simulink model "s_cd_hmc_v3_pol0"  (R2016b)
(part 2 of 31)

      | port_label('output', 1, 'q');
      | disp(['Z^-', num2str(latency)]);
  pipeline92 : Subsystem  AncestorBlock=casper_library_delays/pipeline  mask(pipeline){latency=1}
      mask help:
      | An explicitly laid-out delay line to avoid mapping to SRL16s
      | for use in pipelining to help achieve timing closure.
      mask init:
      | pipeline_init(gcb,'latency',latency);
      settings: AttributesFormatString=Latency = %<latency>
      mask Display:
      | port_label('input', 1, 'd');
      | port_label('output', 1, 'q');
      | disp(['Z^-', num2str(latency)]);
  pipeline93 : Subsystem  AncestorBlock=casper_library_delays/pipeline  mask(pipeline){latency=1}
      mask help:
      | An explicitly laid-out delay line to avoid mapping to SRL16s
      | for use in pipelining to help achieve timing closure.
      mask init:
      | pipeline_init(gcb,'latency',latency);
      settings: AttributesFormatString=Latency = %<latency>
      mask Display:
      | port_label('input', 1, 'd');
      | port_label('output', 1, 'q');
      | disp(['Z^-', num2str(latency)]);
  pipeline94 : Subsystem  AncestorBlock=casper_library_delays/pipeline  mask(pipeline){latency=1}
      mask help:
      | An explicitly laid-out delay line to avoid mapping to SRL16s
      | for use in pipelining to help achieve timing closure.
      mask init:
      | pipeline_init(gcb,'latency',latency);
      settings: AttributesFormatString=Latency = %<latency>
      mask Display:
      | port_label('input', 1, 'd');
      | port_label('output', 1, 'q');
      | disp(['Z^-', num2str(latency)]);
  pipeline95 : Subsystem  AncestorBlock=casper_library_delays/pipeline  mask(pipeline){latency=1}
      mask help:
      | An explicitly laid-out delay line to avoid mapping to SRL16s
      | for use in pipelining to help achieve timing closure.
      mask init:
      | pipeline_init(gcb,'latency',latency);
      settings: AttributesFormatString=Latency = %<latency>
      mask Display:
      | port_label('input', 1, 'd');
      | port_label('output', 1, 'q');
      | disp(['Z^-', num2str(latency)]);
  pipeline96 : Subsystem  AncestorBlock=casper_library_delays/pipeline  mask(pipeline){latency=1}
      mask help:
      | An explicitly laid-out delay line to avoid mapping to SRL16s
      | for use in pipelining to help achieve timing closure.
      mask init:
      | pipeline_init(gcb,'latency',latency);
      settings: AttributesFormatString=Latency = %<latency>
      mask Display:
      | port_label('input', 1, 'd');
      | port_label('output', 1, 'q');
      | disp(['Z^-', num2str(latency)]);
  pipeline97 : Subsystem  AncestorBlock=casper_library_delays/pipeline  mask(pipeline){latency=1}
      mask help:
      | An explicitly laid-out delay line to avoid mapping to SRL16s
      | for use in pipelining to help achieve timing closure.
      mask init:
      | pipeline_init(gcb,'latency',latency);
      settings: AttributesFormatString=Latency = %<latency>
      mask Display:
      | port_label('input', 1, 'd');
      | port_label('output', 1, 'q');
      | disp(['Z^-', num2str(latency)]);
  pipeline98 : Subsystem  AncestorBlock=casper_library_delays/pipeline  mask(pipeline){latency=1}
      mask help:
      | An explicitly laid-out delay line to avoid mapping to SRL16s
      | for use in pipelining to help achieve timing closure.
      mask init:
      | pipeline_init(gcb,'latency',latency);
      settings: AttributesFormatString=Latency = %<latency>
      mask Display:
      | port_label('input', 1, 'd');
      | port_label('output', 1, 'q');
      | disp(['Z^-', num2str(latency)]);
  pipeline99 : Subsystem  AncestorBlock=casper_library_delays/pipeline  mask(pipeline){latency=2}
      mask help:
      | An explicitly laid-out delay line to avoid mapping to SRL16s
      | for use in pipelining to help achieve timing closure.
      mask init:
      | pipeline_init(gcb,'latency',latency);
      settings: AttributesFormatString=Latency = %<latency>
      mask Display:
      | port_label('input', 1, 'd');
      | port_label('output', 1, 'q');
      | disp(['Z^-', num2str(latency)]);
  port0 : Subsystem  Tag=xps:sw_reg  AncestorBlock=xps_library/software register  mask(swreg){io_dir=From Processor, io_delay=0, sample_period=1, names=reg, bitwidths=32, bin_pts=0, arith_types=0, sim_port=on, show_format=on}
      mask prompts: io_dir "I/O direction"; io_delay "I/O delay"; sample_period "Sample period"; names "Bitfield names [msb...lsb]"; bitwidths "Bitfield widths"; bin_pts "Bitfield binary pts"; arith_types "Bitfield types, ufix=0, fix=1, bool=2"; sim_port "Provide sim input/output?"; show_format "Print format string?"
      mask help: A 32-bit software-accessible register. Can be divided into bitfields of varying widths and types using the fields in the block mask.
      mask init:
      | swreg_init(gcb)
      settings: AttributesFormatString=1input:uf32.0 = 32 bits
      mask TypeOptions io_dir: To Processor | From Processor
      mask Callback io_dir:
      | mask_enables = get_param(gcb, 'MaskEnables');
      | mask_names = get_param(gcb, 'MaskNames');
      | if strcmp(get_param(gcb, 'io_dir'), 'To Processor'),
      |     mask_enables{ismember(mask_names, 'sample_period')} = 'off';
      | else
      |     mask_enables{ismember(mask_names, 'sample_period')} = 'on';
      | end
      | set_param(gcb, 'MaskEnables', mask_enables);
  sync : Subsystem  Tag=xps:sw_reg  AncestorBlock=xps_library/software_register  mask(swreg){io_dir=To Processor, io_delay=0, sample_period=1, names=reg, bitwidths=1, bin_pts=0, arith_types=2, sim_port=on, show_format=on}
      mask prompts: io_dir "I/O direction"; io_delay "I/O delay"; sample_period "Sample period"; names "Bitfield names [msb...lsb]"; bitwidths "Bitfield widths"; bin_pts "Bitfield binary pts"; arith_types "Bitfield types, ufix=0, fix=1, bool=2"; sim_port "Provide sim input/output?"; show_format "Print format string?"
      mask help: A 32-bit software-accessible register. Can be divided into bitfields of varying widths and types using the fields in the block mask.
      mask init:
      | swreg_init(gcb)
      settings: AttributesFormatString=1output:b = 1 bits
      mask TypeOptions io_dir: To Processor | From Processor
      mask Callback io_dir:
      | mask_enables = get_param(gcb, 'MaskEnables');
      | mask_names = get_param(gcb, 'MaskNames');
      | if strcmp(get_param(gcb, 'io_dir'), 'To Processor'),
      |     mask_enables{ismember(mask_names, 'sample_period')} = 'off';
      | else
      |     mask_enables{ismember(mask_names, 'sample_period')} = 'on';
      | end
      | set_param(gcb, 'MaskEnables', mask_enables);
  sync_cnt : Subsystem  Tag=xps:sw_reg  AncestorBlock=xps_library/software_register  mask(swreg){io_dir=To Processor, io_delay=0, sample_period=1, names=reg, bitwidths=32, bin_pts=0, arith_types=0, sim_port=on, show_format=on}
      mask prompts: io_dir "I/O direction"; io_delay "I/O delay"; sample_period "Sample period"; names "Bitfield names [msb...lsb]"; bitwidths "Bitfield widths"; bin_pts "Bitfield binary pts"; arith_types "Bitfield types, ufix=0, fix=1, bool=2"; sim_port "Provide sim input/output?"; show_format "Print format string?"
      mask help: A 32-bit software-accessible register. Can be divided into bitfields of varying widths and types using the fields in the block mask.
      mask init:
      | swreg_init(gcb)
      settings: AttributesFormatString=1output:uf32.0 = 32 bits
      mask TypeOptions io_dir: To Processor | From Processor
      mask Callback io_dir:
      | mask_enables = get_param(gcb, 'MaskEnables');
      | mask_names = get_param(gcb, 'MaskNames');
      | if strcmp(get_param(gcb, 'io_dir'), 'To Processor'),
      |     mask_enables{ismember(mask_names, 'sample_period')} = 'off';
      | else
      |     mask_enables{ismember(mask_names, 'sample_period')} = 'on';
      | end
      | set_param(gcb, 'MaskEnables', mask_enables);
  sync_select : Subsystem  Tag=xps:sw_reg  AncestorBlock=xps_library/software register  mask(swreg){io_dir=From Processor, io_delay=0, sample_period=1, names=reg, bitwidths=2, bin_pts=0, arith_types=0, sim_port=on, show_format=on}
      mask prompts: io_dir "I/O direction"; io_delay "I/O delay"; sample_period "Sample period"; names "Bitfield names [msb...lsb]"; bitwidths "Bitfield widths"; bin_pts "Bitfield binary pts"; arith_types "Bitfield types, ufix=0, fix=1, bool=2"; sim_port "Provide sim input/output?"; show_format "Print format string?"
      mask help: A 32-bit software-accessible register. Can be divided into bitfields of varying widths and types using the fields in the block mask.
      mask init:
      | swreg_init(gcb)
      settings: AttributesFormatString=1input:uf2.0 = 2 bits
      mask TypeOptions io_dir: To Processor | From Processor
      mask Callback io_dir:
      | mask_enables = get_param(gcb, 'MaskEnables');
      | mask_names = get_param(gcb, 'MaskNames');
      | if strcmp(get_param(gcb, 'io_dir'), 'To Processor'),
      |     mask_enables{ismember(mask_names, 'sample_period')} = 'off';
      | else
      |     mask_enables{ismember(mask_names, 'sample_period')} = 'on';
      | end
      | set_param(gcb, 'MaskEnables', mask_enables);
  time_gen_cd : Subsystem  mask{n_bits_period=fft_stages-1-2, n_bits_increment=0, n_bits_counter=48-fft_stages}
      mask prompts: n_bits_period "Period (2^?)"; n_bits_increment "Increment (2^?)"; n_bits_counter "Counter size (2^?)"
  tl_cd0 : Subsystem  mask(timed_latch){n_bits_time=48-fft_stages, n_bits_quantization=fft_stages, n_bits_counters=4}
      mask prompts: n_bits_time "Number bits in time to compare"; n_bits_quantization "Time offset from lsb"; n_bits_counters "Bits in status counters"
      mask help:
      | Latches load_value when armed and current_time matches requested time.
      | current_time should be in ADC samples.
      mask init:
      | set_param([gcb,'/status'], 'bitwidths', mat2str([1, repmat(n_bits_counters, 1, 2)]));
      mask Help:
      | When armed, will latch new value when current time matches the time
      | specified. The input time should be in samples and mask settings allow
      | a portion of this to be compared to cater for quantization. Arm and latch
      | counts allow the current state, pending and missed latch events to be
      | determined.
  tl_cd0_control : Subsystem  Tag=xps:sw_reg  AncestorBlock=xps_library/software_register  mask(swreg){io_dir=From Processor, io_delay=0, sample_period=1, names=[arm load_immediate load_time_msw], bitwidths=[1 1 16], bin_pts=[0 0 0], arith_types=[2 2 0], sim_port=on, show_format=on}
      mask prompts: io_dir "I/O direction"; io_delay "I/O delay"; sample_period "Sample period"; names "Bitfield names [msb...lsb]"; bitwidths "Bitfield widths"; bin_pts "Bitfield binary pts"; arith_types "Bitfield types, ufix=0, fix=1, bool=2"; sim_port "Provide sim input/output?"; show_format "Print format string?"
      mask help: A 32-bit software-accessible register. Can be divided into bitfields of varying widths and types using the fields in the block mask.
      mask init:
      | swreg_init(gcb)
      settings: AttributesFormatString=3 inputs:b,b,uf16.0 = 18 bits
      mask TypeOptions io_dir: To Processor | From Processor
      mask Callback io_dir:
      | mask_enables = get_param(gcb, 'MaskEnables');
      | mask_names = get_param(gcb, 'MaskNames');
      | if strcmp(get_param(gcb, 'io_dir'), 'To Processor'),
      |     mask_enables{ismember(mask_names, 'sample_period')} = 'off';
      | else
      |     mask_enables{ismember(mask_names, 'sample_period')} = 'on';
      | end
      | set_param(gcb, 'MaskEnables', mask_enables);
  tl_cd0_control_lsw : Subsystem  Tag=xps:sw_reg  AncestorBlock=xps_library/software_register  mask(swreg){io_dir=From Processor, io_delay=0, sample_period=1, names=load_time_lsw, bitwidths=32, bin_pts=0, arith_types=0, sim_port=on, show_format=on}
      mask prompts: io_dir "I/O direction"; io_delay "I/O delay"; sample_period "Sample period"; names "Bitfield names [msb...lsb]"; bitwidths "Bitfield widths"; bin_pts "Bitfield binary pts"; arith_types "Bitfield types, ufix=0, fix=1, bool=2"; sim_port "Provide sim input/output?"; show_format "Print format string?"
      mask help: A 32-bit software-accessible register. Can be divided into bitfields of varying widths and types using the fields in the block mask.
      mask init:
      | swreg_init(gcb)
      settings: AttributesFormatString=1input:uf32.0 = 32 bits
      mask TypeOptions io_dir: To Processor | From Processor
      mask Callback io_dir:
      | mask_enables = get_param(gcb, 'MaskEnables');
      | mask_names = get_param(gcb, 'MaskNames');
      | if strcmp(get_param(gcb, 'io_dir'), 'To Processor'),
      |     mask_enables{ismember(mask_names, 'sample_period')} = 'off';
      | else
      |     mask_enables{ismember(mask_names, 'sample_period')} = 'on';
      | end
      | set_param(gcb, 'MaskEnables', mask_enables);
  tl_cd1_control : Subsystem  Tag=xps:sw_reg  AncestorBlock=xps_library/software_register  mask(swreg){io_dir=From Processor, io_delay=0, sample_period=1, names=[arm load_immediate load_time_msw], bitwidths=[1 1 16], bin_pts=[0 0 0], arith_types=[2 2 0], sim_port=on, show_format=on}
      mask prompts: io_dir "I/O direction"; io_delay "I/O delay"; sample_period "Sample period"; names "Bitfield names [msb...lsb]"; bitwidths "Bitfield widths"; bin_pts "Bitfield binary pts"; arith_types "Bitfield types, ufix=0, fix=1, bool=2"; sim_port "Provide sim input/output?"; show_format "Print format string?"
      mask help: A 32-bit software-accessible register. Can be divided into bitfields of varying widths and types using the fields in the block mask.
      mask init:
      | swreg_init(gcb)
      settings: AttributesFormatString=3 inputs:b,b,uf16.0 = 18 bits
      mask TypeOptions io_dir: To Processor | From Processor
      mask Callback io_dir:
      | mask_enables = get_param(gcb, 'MaskEnables');
      | mask_names = get_param(gcb, 'MaskNames');
      | if strcmp(get_param(gcb, 'io_dir'), 'To Processor'),
      |     mask_enables{ismember(mask_names, 'sample_period')} = 'off';
      | else
      |     mask_enables{ismember(mask_names, 'sample_period')} = 'on';
      | end
      | set_param(gcb, 'MaskEnables', mask_enables);
  tl_cd1_control_lsw : Subsystem  Tag=xps:sw_reg  AncestorBlock=xps_library/software_register  mask(swreg){io_dir=From Processor, io_delay=0, sample_period=1, names=load_time_lsw, bitwidths=32, bin_pts=0, arith_types=0, sim_port=on, show_format=on}
      mask prompts: io_dir "I/O direction"; io_delay "I/O delay"; sample_period "Sample period"; names "Bitfield names [msb...lsb]"; bitwidths "Bitfield widths"; bin_pts "Bitfield binary pts"; arith_types "Bitfield types, ufix=0, fix=1, bool=2"; sim_port "Provide sim input/output?"; show_format "Print format string?"
      mask help: A 32-bit software-accessible register. Can be divided into bitfields of varying widths and types using the fields in the block mask.
      mask init:
      | swreg_init(gcb)
      settings: AttributesFormatString=1input:uf32.0 = 32 bits
      mask TypeOptions io_dir: To Processor | From Processor
      mask Callback io_dir:
      | mask_enables = get_param(gcb, 'MaskEnables');
      | mask_names = get_param(gcb, 'MaskNames');
      | if strcmp(get_param(gcb, 'io_dir'), 'To Processor'),
      |     mask_enables{ismember(mask_names, 'sample_period')} = 'off';
      | else
      |     mask_enables{ismember(mask_names, 'sample_period')} = 'on';
      | end
      | set_param(gcb, 'MaskEnables', mask_enables);
  tl_cd_bs0 : Subsystem  mask(timed_latch){n_bits_time=48-fft_stages, n_bits_quantization=fft_stages, n_bits_counters=4}
      mask prompts: n_bits_time "Number bits in time to compare"; n_bits_quantization "Time offset from lsb"; n_bits_counters "Bits in status counters"
      mask help:
      | Latches load_value when armed and current_time matches requested time.
      | current_time should be in ADC samples.
      mask init:
      | set_param([gcb,'/status'], 'bitwidths', mat2str([1, repmat(n_bits_counters, 1, 2)]));
      mask Help:
      | When armed, will latch new value when current time matches the time
      | specified. The input time should be in samples and mask settings allow
      | a portion of this to be compared to cater for quantization. Arm and latch
      | counts allow the current state, pending and missed latch events to be
      | determined.
  tx_metadata : Subsystem  Tag=xps:sw_reg  AncestorBlock=xps_library/software register  mask(swreg){io_dir=From Processor, io_delay=0, sample_period=1, names=[porttx board_id], bitwidths=16, bin_pts=0, arith_types=0, sim_port=on, show_format=on}
      mask prompts: io_dir "I/O direction"; io_delay "I/O delay"; sample_period "Sample period"; names "Bitfield names [msb...lsb]"; bitwidths "Bitfield widths"; bin_pts "Bitfield binary pts"; arith_types "Bitfield types, ufix=0, fix=1, bool=2"; sim_port "Provide sim input/output?"; show_format "Print format string?"
      mask help: A 32-bit software-accessible register. Can be divided into bitfields of varying widths and types using the fields in the block mask.
      mask init:
      | swreg_init(gcb)
      settings: AttributesFormatString=2 inputs:uf16.0,uf16.0 = 32 bits
      mask TypeOptions io_dir: To Processor | From Processor
      mask Callback io_dir:
      | mask_enables = get_param(gcb, 'MaskEnables');
      | mask_names = get_param(gcb, 'MaskNames');
      | if strcmp(get_param(gcb, 'io_dir'), 'To Processor'),
      |     mask_enables{ismember(mask_names, 'sample_period')} = 'off';
      | else
      |     mask_enables{ismember(mask_names, 'sample_period')} = 'on';
      | end
      | set_param(gcb, 'MaskEnables', mask_enables);
  valid80 : Subsystem  Tag=xps:sw_reg  AncestorBlock=xps_library/software_register  mask(swreg){io_dir=To Processor, io_delay=0, sample_period=1, names=reg, bitwidths=1, bin_pts=0, arith_types=2, sim_port=on, show_format=on}
      mask prompts: io_dir "I/O direction"; io_delay "I/O delay"; sample_period "Sample period"; names "Bitfield names [msb...lsb]"; bitwidths "Bitfield widths"; bin_pts "Bitfield binary pts"; arith_types "Bitfield types, ufix=0, fix=1, bool=2"; sim_port "Provide sim input/output?"; show_format "Print format string?"
      mask help: A 32-bit software-accessible register. Can be divided into bitfields of varying widths and types using the fields in the block mask.
      mask init:
      | swreg_init(gcb)
      settings: AttributesFormatString=1output:b = 1 bits
      mask TypeOptions io_dir: To Processor | From Processor
      mask Callback io_dir:
      | mask_enables = get_param(gcb, 'MaskEnables');
      | mask_names = get_param(gcb, 'MaskNames');
      | if strcmp(get_param(gcb, 'io_dir'), 'To Processor'),
      |     mask_enables{ismember(mask_names, 'sample_period')} = 'off';
      | else
      |     mask_enables{ismember(mask_names, 'sample_period')} = 'on';
      | end
      | set_param(gcb, 'MaskEnables', mask_enables);
  valid80_cnt : Subsystem  Tag=xps:sw_reg  AncestorBlock=xps_library/software_register  mask(swreg){io_dir=To Processor, io_delay=0, sample_period=1, names=reg, bitwidths=32, bin_pts=0, arith_types=0, sim_port=on, show_format=on}
      mask prompts: io_dir "I/O direction"; io_delay "I/O delay"; sample_period "Sample period"; names "Bitfield names [msb...lsb]"; bitwidths "Bitfield widths"; bin_pts "Bitfield binary pts"; arith_types "Bitfield types, ufix=0, fix=1, bool=2"; sim_port "Provide sim input/output?"; show_format "Print format string?"
      mask help: A 32-bit software-accessible register. Can be divided into bitfields of varying widths and types using the fields in the block mask.
      mask init:
      | swreg_init(gcb)
      settings: AttributesFormatString=1output:uf32.0 = 32 bits
      mask TypeOptions io_dir: To Processor | From Processor
      mask Callback io_dir:
      | mask_enables = get_param(gcb, 'MaskEnables');
      | mask_names = get_param(gcb, 'MaskNames');
      | if strcmp(get_param(gcb, 'io_dir'), 'To Processor'),
      |     mask_enables{ismember(mask_names, 'sample_period')} = 'off';
      | else
      |     mask_enables{ismember(mask_names, 'sample_period')} = 'on';
      | end
      | set_param(gcb, 'MaskEnables', mask_enables);
  wb_prog_delay : Subsystem  mask{n_bits_fft=fft_stages, n_bits_cd=17}
      mask prompts: n_bits_fft "fft length (2^?)"; n_bits_cd "max coarse delay (2^?)"
  tag scope: addr_map_sel=global, cnt_rst=global, dvalid=global, sync_select=global, sys_rst=global
  wires:
  Constant/1 -> port0/1(sim_1)
  port0/1(in_reg) -> Delay16/1
  Constant2/1 -> ip0/1(sim_1)
  ip0/1(in_reg) -> Delay15/1
  Constant3/1 -> forty_gbe/8(rx_overrun_ack)
  Constant4/1 -> forty_gbe/7(rx_ack)
  [gbe_rst] -> pipeline102/1(d)
  Delay15/1 -> forty_gbe/4(tx_dest_ip)
  Delay16/1 -> forty_gbe/5(tx_dest_port)
  Concat22/1 -> pipeline29/1(d)
  Concat3/1 -> pipeline27/1(d)
  phase0/1(in_initial) -> Reinterpret2/1
  delta_delay0/1(in_delta) -> Reinterpret1/1
  phase0/2(in_delta) -> Reinterpret3/1
  Reinterpret8/1 -> pipeline56/1(d)
  Reinterpret1/1 -> pipeline55/1(d)
  Reinterpret2/1 -> pipeline54/1(d)
  Reinterpret3/1 -> pipeline53/1(d)
  phase1/1(in_initial) -> Reinterpret5/1
  delta_delay1/1(in_delta) -> Reinterpret4/1
  phase1/2(in_delta) -> Reinterpret6/1
  Reinterpret4/1 -> pipeline51/1(d)
  Reinterpret5/1 -> pipeline50/1(d)
  Reinterpret6/1 -> pipeline49/1(d)
  Reinterpret7/1 -> pipeline52/1(d)
  delay0/1(in_initial) -> Reinterpret8/1
  delay1/1(in_initial) -> Reinterpret7/1
  Constant10/1 -> iptx_base/1(sim_1)
  Constant9/1 -> tx_metadata/1(sim_1)
  Constant13/1 -> tx_metadata/2(sim_2)
  iptx_base/1(in_reg) -> pipeline105/1(d)
  pipeline105/1(q) -> [tx_ip_base]
  tx_metadata/1(in_porttx) -> pipeline106/1(d)
  tx_metadata/2(in_board_id) -> pipeline107/1(d)
  pipeline106/1(q) -> [tx_port]
  pipeline107/1(q) -> [tx_board_id]
  edge_detect4/1(out) -> pipeline5/1(d)
  control/6(in_cnt_rst) -> edge_detect1/1(in)
  edge_detect1/1(out) -> pipeline14/1(d)
  control/3(in_gbe_rst) -> pipeline6/1(d)
  control/1(in_sys_rst) -> edge_detect7/1(in)
  pipeline3/1(q) -> [sys_rst]
  pipeline5/1(q) -> [clr_status]
  pipeline6/1(q) -> [gbe_rst]
  pipeline7/1(q) -> [gbe_txen]
  pipeline13/1(q) -> [tvg_adc_en]
  pipeline14/1(q) -> [cnt_rst]
  control/5(in_tvg_adc) -> pipeline13/1(d)
  edge_detect2/1(out) -> pipeline38/1(d)
  pipeline38/1(q) -> [gbe_cnt_rst]
  control/7(in_gbe_cnt_rst) -> edge_detect2/1(in)
  control/4(in_gbe_txen) -> pipeline7/1(d)
  control/2(in_status_clr) -> edge_detect4/1(in)
  pipeline43/1(q) -> [adc_snap_arm]
  control/8(in_adc_snap_arm) -> pipeline43/1(d)
  control/9(in_adc_snap_trig_select) -> pipeline39/1(d)
  pipeline39/1(q) -> [adc_snap_trig_source]
  Counter2/1 -> pipeline31/1(d)
  Counter4/1 -> pipeline32/1(d)
  Counter9/1 -> pipeline33/1(d)
  Counter10/1 -> pipeline34/1(d)
  Counter11/1 -> pipeline35/1(d)
  Counter12/1 -> pipeline36/1(d)
  Counter14/1 -> pipeline40/1(d)
  Counter13/1 -> pipeline37/1(d)
  hmc_error/1(sim_out) -> Terminator9/1
  [hmc_error] -> hmc_error/1(out_reg)
  hmc_parity/1(sim_out) -> Terminator11/1
  [hmc_parity_pol0] -> hmc_parity/1(out_reg)
  Constant11/1 -> Delay10/1
  [valid80_local] -> Gateway Out19/1, pipeline58/1(d), pipeline61/1(d), pipeline62/1(d), pipeline63/1(d), pipeline64/1(d), pipeline65/1(d), pipeline66/1(d), pipeline60/1(d), pipeline59/1(d)
  bus_create1/1(bus_out) -> [cd_in]
  pipeline30/1(q) -> [valid80_cd]
  Constant24/1 -> forty_gbe/2(tx_data)
  Constant25/1 -> forty_gbe/3(tx_valid)
  Constant26/1 -> forty_gbe/6(tx_end_of_frame)
  pipeline27/1(q) -> [ld_val1]
  pipeline29/1(q) -> [ld_val0]
  pipeline49/1(q) -> Concat3/4
  pipeline50/1(q) -> Concat3/3
  pipeline51/1(q) -> Concat3/2
  pipeline52/1(q) -> Concat3/1
  pipeline53/1(q) -> Concat22/4
  pipeline54/1(q) -> Concat22/3
  pipeline55/1(q) -> Concat22/2
  pipeline56/1(q) -> Concat22/1
  bus_expand2/1(msb_out8) -> pipeline167/1(d)  "hmc_out9"
  bus_expand2/8(lsb_out1) -> pipeline73/1(d)  "hmc_out16"
  pipeline73/1(q) -> hmc_out/8(in_d07)
  pipeline72/1(q) -> hmc_out/7(in_d06)
  pipeline71/1(q) -> hmc_out/6(in_d05)
  pipeline70/1(q) -> hmc_out/5(in_d04)
  pipeline69/1(q) -> hmc_out/4(in_d03)
  pipeline68/1(q) -> hmc_out/3(in_d02)
  pipeline67/1(q) -> hmc_out/2(in_d01)
  pipeline167/1(q) -> hmc_out/1(in_d00)
  bus_expand2/7(out2) -> pipeline72/1(d)
  bus_expand2/5(out4) -> pipeline70/1(d)
  bus_expand2/4(out5) -> pipeline69/1(d)
  bus_expand2/6(out3) -> pipeline71/1(d)
  bus_expand2/3(out6) -> pipeline68/1(d)
  bus_expand2/2(out7) -> pipeline67/1(d)
  pipeline75/1(q) -> hmc_out/9(in_dvalid)
  pipeline74/1(q) -> hmc_out/10(in_sync)
  pipeline65/1(q) -> Counter14/2
  pipeline64/1(q) -> Counter13/2
  pipeline63/1(q) -> Counter12/2
  pipeline62/1(q) -> Counter11/2
  pipeline61/1(q) -> Counter10/2
  pipeline59/1(q) -> Counter4/2
  pipeline60/1(q) -> Counter9/2
  pipeline58/1(q) -> Counter2/2
  pipeline98/1(q) -> Counter2/1
  pipeline97/1(q) -> Counter4/1
  pipeline96/1(q) -> Counter9/1
  pipeline95/1(q) -> Counter10/1
  pipeline94/1(q) -> Counter11/1
  pipeline93/1(q) -> Counter12/1
  pipeline92/1(q) -> Counter13/1
  pipeline91/1(q) -> Counter14/1
  hmc_delay/1(sim_out) -> Terminator/1
  compute_delay/1(hmc_latency) -> pipeline99/1(d)
  pipeline99/1(q) -> hmc_delay/1(out_reg)
  pipeline102/1(q) -> forty_gbe/1(rst)
  [cd_in] -> pipeline108/1(d)
  [hmc_data_p0] -> pipeline111/1(d)
  [hmc_dvalid_p0] -> pipeline110/1(d)
  [hmc_sync_p0] -> pipeline109/1(d)
  Constant1/1 -> pipeline112/1(d)
  [valid80_cd] -> pipeline104/1(d)
  [sync80_cd] -> pipeline103/1(d)
  pipeline103/1(q) -> compute_delay/1(cd_in_sync)
  pipeline104/1(q) -> compute_delay/2(cd_in_dvalid)
  pipeline108/1(q) -> compute_delay/3(cd_in)
  pipeline109/1(q) -> compute_delay/4(cd_out_sync)
  pipeline110/1(q) -> compute_delay/5(cd_out_dvalid)
  pipeline111/1(q) -> compute_delay/6(cd_out)
  pipeline112/1(q) -> compute_delay/7(trigger_threshold)
  cd_in_cnt_thresh/1(sim_out) -> Terminator2/1
  pipeline113/1(q) -> cd_in_cnt_thresh/1(out_reg)
  cd_out_cnt_thresh/1(sim_out) -> Terminator3/1
  pipeline114/1(q) -> cd_out_cnt_thresh/1(out_reg)
  compute_delay/3(cd_out_count_sync_threshold) -> pipeline114/1(d)
  compute_delay/2(cd_in_count_sync_threshold) -> pipeline113/1(d)
  Constant5/1 -> sync_select/1(sim_1)
  pipeline2/1(q) -> bus_expand3/1(bus_in)
  [cd_in] -> pipeline2/1(d)
  Gateway Out45/1 -> To Workspace2/1
  Gateway Out46/1 -> To Workspace3/1
  Gateway Out47/1 -> To Workspace5/1
  Gateway Out48/1 -> To Workspace11/1
  Gateway Out49/1 -> To Workspace12/1
  Gateway Out50/1 -> To Workspace13/1
  Gateway Out51/1 -> To Workspace14/1
  bus_expand3/1(msb_out8) -> Gateway Out43/1
  bus_expand3/2(out7) -> Gateway Out45/1
  bus_expand3/3(out6) -> Gateway Out46/1
  bus_expand3/4(out5) -> Gateway Out47/1
  bus_expand3/5(out4) -> Gateway Out48/1
  bus_expand3/6(out3) -> Gateway Out49/1
  bus_expand3/7(out2) -> Gateway Out50/1
  bus_expand3/8(lsb_out1) -> Gateway Out51/1
  Gateway Out43/1 -> To Workspace4/1
  [hmc_data_p0] -> bus_expand4/1(bus_in)
  Gateway Out3/1 -> To Workspace16/1
  Gateway Out5/1 -> To Workspace17/1
  Gateway Out6/1 -> To Workspace18/1
  Gateway Out7/1 -> To Workspace19/1
  bus_expand4/1(msb_out8) -> Gateway Out2/1
  bus_expand4/2(out7) -> Gateway Out3/1
  bus_expand4/3(out6) -> Gateway Out5/1
  bus_expand4/4(out5) -> Gateway Out6/1
  bus_expand4/5(out4) -> Gateway Out7/1
  bus_expand4/6(out3) -> Gateway Out8/1
  bus_expand4/7(out2) -> Gateway Out9/1
  bus_expand4/8(lsb_out1) -> Gateway Out12/1
  Gateway Out2/1 -> To Workspace21/1
  Gateway Out12/1 -> To Workspace23/1
  Gateway Out9/1 -> To Workspace22/1
  Gateway Out8/1 -> To Workspace20/1
  [sync80_local] -> Gateway Out18/1, pipeline8/1(d)
  pipeline9/1(q) -> [sync80_cd]
  Gateway Out18/1 -> To Workspace26/1
  Gateway Out19/1 -> To Workspace27/1
  sync_select/1(in_reg) -> pipeline4/1(d)
  pipeline4/1(q) -> [sync_select]
  dvalid/1(in_reg) -> pipeline16/1(d)
  pipeline16/1(q) -> [dvalid]
  man_sync/1(in_reg) -> pipeline17/1(d)
  Constant17/1 -> Delay/1
  sync/1(sim_out) -> To Workspace102/1
  edge_detect9/1 -> Register1/3, Register1/1, Counter1/2
  sync_cnt/1(sim_out) -> To Workspace104/1
  Counter1/1 -> pipeline129/1(d)
  pipeline129/1(q) -> sync_cnt/1(out_reg)
  pipeline131/1(q) -> sync/1(out_reg)
  Register1/1 -> pipeline131/1(d)
  [sys_rst] -> edge_detect11/1
  [sync80_local] -> edge_detect9/1
  valid80/1(sim_out) -> To Workspace38/1
  edge_detect5/1 -> Register2/3, Register2/1, Counter3/2
  valid80_cnt/1(sim_out) -> To Workspace39/1
  Counter3/1 -> pipeline28/1(d)
  pipeline28/1(q) -> valid80_cnt/1(out_reg)
  pipeline44/1(q) -> valid80/1(out_reg)
  Register2/1 -> pipeline44/1(d)
  [sys_rst] -> edge_detect6/1
  [valid80_local] -> edge_detect5/1
  pipeline17/1(q) -> [man_sync]
  Delay/1 -> man_sync/1(sim_1)
  Delay10/1 -> dvalid/1(sim_1)
  bus_expand1/8(lsb_out1) -> pipeline176/1(d)  "hmc_out16"
  pipeline222/1(q) -> bus_expand1/1(bus_in)
  [cd_in] -> pipeline222/1(d)
  pipeline176/1(q) -> cd_in/8(in_d07)
  pipeline175/1(q) -> cd_in/7(in_d06)
  pipeline172/1(q) -> cd_in/6(in_d05)
  pipeline171/1(q) -> cd_in/5(in_d04)
  pipeline170/1(q) -> cd_in/4(in_d03)
  pipeline169/1(q) -> cd_in/3(in_d02)
  pipeline168/1(q) -> cd_in/2(in_d01)
  bus_expand1/7(out2) -> pipeline175/1(d)
  bus_expand1/5(out4) -> pipeline171/1(d)
  bus_expand1/4(out5) -> pipeline170/1(d)
  bus_expand1/6(out3) -> pipeline172/1(d)
  bus_expand1/3(out6) -> pipeline169/1(d)
  bus_expand1/2(out7) -> pipeline168/1(d)
  pipeline19/1(q) -> pipeline178/1(d), Logical/1
  pipeline178/1(q) -> cd_in/9(in_dvalid)
  pipeline177/1(q) -> cd_in/10(in_sync)
  bus_expand1/1(msb_out8) -> pipeline87/1(d)
  pipeline87/1(q) -> cd_in/1(in_d00)
  [valid80_cd] -> pipeline19/1(d)
  [sync80_cd] -> pipeline15/1(d)
  pipeline15/1(q) -> pipeline177/1(d), pipeline57/1(d), Logical/2
  pipeline57/1(q) -> cd_in/12(trig)
  pipeline18/1(q) -> cd_in/11(we)
  Logical/1 -> pipeline18/1(d)
  pipeline81/1(q) -> hmc_out/12(trig)
  pipeline78/1(q) -> hmc_out/11(we)
  Logical1/1 -> pipeline78/1(d)
  [hmc_sync_p0] -> pipeline81/1(d), Logical1/2, pipeline74/1(d)
  Counter5/1 -> Gateway Out27/1, Relational1/1
  Constant32/1 -> Relational1/2
  Gateway Out15/1 -> To Workspace42/1
  Gateway Out1/1 -> To Workspace1/1
  Delay1/1 -> Delay3/1
  Delay7/1 -> Delay12/1
  Gateway Out4/1 -> To Workspace10/1
  Delay9/1 -> Delay13/1
  [valid80] -> Terminator1/1
  Mux1/1 -> edge_detect12/1
  Delay3/1 -> Gateway Out28/1, Mux2/2
  [sync_select] -> Mux2/1, Gateway Out25/1, Mux1/1
  [dvalid] -> Logical16/3
  Register3/1 -> Delay8/1, Gateway Out29/1, Inverter3/1
  Delay6/1 -> Delay17/1
  Delay8/1 -> Delay1/1
  Gateway Out24/1 -> To Workspace35/1
  Gateway Out25/1 -> To Workspace36/1
  Gateway Out26/1 -> To Workspace37/1
  Gateway Out27/1 -> To Workspace40/1
  Register4/1 -> Delay7/1, Delay5/1, Delay2/1, Logical2/1
  Mux2/1 -> Delay14/1
  Gateway Out28/1 -> To Workspace41/1
  Delay4/1 -> Mux2/3
  Relational1/1 -> Mux1/3, Gateway Out24/1
  Delay17/1 -> Gateway Out26/1, Mux1/2
  Slice1/1 -> Register3/3, Register3/1, Delay9/1, Gateway Out30/1
  Counter6/1 -> Slice1/1, Gateway Out31/1
  Gateway Out29/1 -> To Workspace9/1
  Gateway Out30/1 -> To Workspace33/1
  Gateway Out31/1 -> To Workspace34/1
  [sys_rst] -> Counter5/1, Counter6/1, Register3/2, Register4/2, Gateway Out33/1
  Inverter3/1 -> Logical2/2
  Logical16/1 -> Register4/3, Delay11/1, Gateway Out32/1, Register4/1
  Gateway Out32/1 -> To Workspace43/1
  Gateway Out33/1 -> To Workspace44/1
  Logical2/1 -> Counter6/2
  Delay2/1 -> Counter5/2
  Delay5/1 -> Relational1/3
  edge_detect12/1 -> [sync80_local], Gateway Out1/1
  [man_sync] -> Mux1/4
  Delay11/1 -> Mux2/4
  [hmc_post] -> Logical16/1
  [hmc_init] -> Logical16/2
  Delay12/1 -> Gateway Out4/1, Delay4/1
  Delay13/1 -> Delay6/1
  pipeline66/1(q) -> pipeline30/1(d)
  pipeline8/1(q) -> pipeline9/1(d)
  Delay14/1 -> [valid80_local], Gateway Out15/1
  pipeline1/1(q) -> [addr_map_sel]
  Constant8/1 -> addr_map_sel/1(sim_1)
  addr_map_sel/1(in_reg) -> pipeline1/1(d)
  edge_detect7/1(out) -> pipeline3/1(d)
  edge_detect11/1 -> Register1/2, Counter1/1
  edge_detect6/1 -> Register2/2, Counter3/1
  Constant7/1 -> delay0/1(sim_1)
  [sync80_local] -> pipeline91/1(d), pipeline92/1(d), pipeline93/1(d), pipeline94/1(d), pipeline95/1(d), pipeline96/1(d), pipeline97/1(d), pipeline98/1(d)
  [hmc_data_p0] -> bus_expand2/1(bus_in)
  [hmc_dvalid_p0] -> pipeline75/1(d), Logical1/1
  cd_compensation0/2(dout) -> [hmc_data_p0]
  cd_compensation0/4(hmc_error) -> [hmc_error]
  [dvalid_tl_cd0] -> Gateway Out42/1, cd_compensation0/3(en)
  [sync_tl_cd0] -> Gateway Out41/1, cd_compensation0/1(sync_in)
  [dout_tl_cd0] -> Gateway Out44/1, cd_compensation0/2(din)
  [en_tl_cd0] -> cd_compensation0/5(load_val)
  [delay_tl_cd0] -> cd_compensation0/4(delay_val)
  Constant33/1 -> time_gen_cd/6(rd_misc_in)
  time_gen_cd/4(rd_misc_out) -> Terminator15/1
  [sync_tl_cd0] -> time_gen_cd/1(wr_sync_in)
  [dvalid_tl_cd0] -> time_gen_cd/2(wr_en)
  [hmc_sync_p0] -> time_gen_cd/4(rd_sync_in)
  [hmc_dvalid_p0] -> time_gen_cd/5(rd_en)
  time_gen_cd/1(rd_sync_out) -> [tg_rd_sync]
  time_gen_cd/2(rd_dvalid) -> [tg_rd_dvalid]
  [dvalid_tl_bs0] -> Gateway Out56/1, wb_prog_delay/4(en)
  [delay_tl_bs0] -> Gateway Out73/1, wb_prog_delay/2(delay_val)
  [delay_tl_sync0] -> Gateway Out55/1, wb_prog_delay/1(sync)
  [en_tl_bs0] -> Gateway Out72/1, wb_prog_delay/5(load_val)
  wb_prog_delay/2(data_out) -> [delay_d0]
  wb_prog_delay/3(dvalid) -> [delay_dv]
  [time80_tl_cd0] -> Slice9/1
  Slice9/1 -> time_gen_cd/3(wr_val_in)
  Constant35/1 -> Concat7/2
  time_gen_cd/3(rd_val_out) -> Concat7/1
  Concat7/1 -> [tg_rd_time_out]
  cd_compensation0/3(dvalid) -> [hmc_dvalid_p0]
  cd_compensation0/1(sync_out) -> [hmc_sync_p0]
  cd_compensation0/5(parity_error) -> [hmc_parity_pol0]
  wb_prog_delay/1(sync_out) -> [delay_sync]
  tl_cd0_control/3(in_load_time_msw) -> Concat6/1
  tl_cd0_control_lsw/1(in_load_time_lsw) -> Concat6/2
  Constant42/1 -> tl_cd0_control_lsw/1(sim_1)
  Constant40/1 -> tl_cd0_control/3(sim_3)
  Constant41/1 -> tl_cd0_control/2(sim_2)
  Constant43/1 -> Delay18/1
  Delay18/1 -> tl_cd0_control/1(sim_1)
  Concat6/1 -> [tl_cd0_load_time]
  tl_cd0_control/2(in_load_immediate) -> [tl_cd0_load_immediate]
  tl_cd0_control/1(in_arm) -> [tl_cd0_arm]
  tl_cd1_control/3(in_load_time_msw) -> Concat8/1
  tl_cd1_control_lsw/1(in_load_time_lsw) -> Concat8/2
  Constant47/1 -> tl_cd1_control_lsw/1(sim_1)
  Constant45/1 -> tl_cd1_control/3(sim_3)
  Constant46/1 -> tl_cd1_control/2(sim_2)
  Constant48/1 -> Delay19/1
  Delay19/1 -> tl_cd1_control/1(sim_1)
  Concat8/1 -> [tl_cd1_load_time]
  tl_cd1_control/2(in_load_immediate) -> [tl_cd1_load_immediate]
  tl_cd1_control/1(in_arm) -> [tl_cd1_arm]
  [ld_val0] -> pipeline20/1(d)
  [clr_status] -> pipeline76/1(d)
  tl_cd0/6(time) -> [time80_tl_cd0]
  Concat1/1 -> Gateway Out40/1, pipeline47/1(d)
  pipeline76/1(q) -> tl_cd0/1(rst)
  pipeline47/1(q) -> tl_cd0/2(current_time)
  pipeline20/1(q) -> tl_cd0/3(load_value)
  pipeline12/1(q) -> tl_cd0/4(sync_in)
  pipeline11/1(q) -> tl_cd0/5(din)
  pipeline77/1(q) -> tl_cd0/6(en)
  [sync80_cd] -> Gateway Out63/1, pipeline12/1(d)
  [valid80_cd] -> Gateway Out62/1, pipeline77/1(d)
  Constant16/1 -> tl_cd0/7(misci)
  tl_cd0/7(misco) -> Terminator5/1
  tl_cd0/3(sync_out) -> [sync_tl_cd0]
  tl_cd0/5(dvalid) -> [dvalid_tl_cd0]
  tl_cd0/4(dout) -> [dout_tl_cd0]
  tl_cd0/2(enable) -> [en_tl_cd0]
  tl_cd0/1(value) -> [delay_tl_cd0]
  pipeline127/1(q) -> tl_cd0/10(load_time)
  pipeline126/1(q) -> tl_cd0/9(load_immediate)
  pipeline125/1(q) -> tl_cd0/8(arm)
  [tl_cd0_arm] -> pipeline125/1(d)
  [tl_cd0_load_immediate] -> pipeline126/1(d)
  [tl_cd0_load_time] -> pipeline127/1(d)
  pipeline101/1(q) -> tl_cd_bs0/1(rst)
  pipeline10/1(q) -> tl_cd_bs0/2(current_time)
  pipeline115/1(q) -> Gateway Out74/1, tl_cd_bs0/3(load_value)
  pipeline116/1(q) -> Gateway Out52/1, tl_cd_bs0/4(sync_in)
  pipeline117/1(q) -> Gateway Out54/1, tl_cd_bs0/5(din)
  pipeline118/1(q) -> Gateway Out53/1, tl_cd_bs0/6(en)
  [clr_status] -> pipeline101/1(d)
  [tg_rd_time_out] -> pipeline10/1(d)
  [ld_val0] -> pipeline115/1(d)
  [tg_rd_sync] -> pipeline116/1(d)
  [tg_rd_dvalid] -> pipeline118/1(d)
  Constant34/1 -> tl_cd_bs0/7(misci)
  tl_cd_bs0/7(misco) -> Terminator12/1
  tl_cd_bs0/4(dout) -> [data_tl_bs0]
  tl_cd_bs0/6(time) -> Terminator13/1
  tl_cd_bs0/5(dvalid) -> [dvalid_tl_bs0]
  tl_cd_bs0/1(value) -> [delay_tl_bs0]
  tl_cd_bs0/3(sync_out) -> [delay_tl_sync0]
  tl_cd_bs0/2(enable) -> [en_tl_bs0]
  pipeline133/1(q) -> tl_cd_bs0/8(arm)
  pipeline134/1(q) -> tl_cd_bs0/9(load_immediate)
  pipeline135/1(q) -> tl_cd_bs0/10(load_time)
  [tl_cd0_arm] -> pipeline133/1(d)
  [tl_cd0_load_immediate] -> pipeline134/1(d)
  [tl_cd0_load_time] -> pipeline135/1(d)
  Gateway Out40/1 -> To Workspace50/1
  Gateway Out38/1 -> To Workspace49/1
  Gateway Out39/1 -> To Workspace28/1
  Gateway Out22/1 -> To Workspace31/1
  Gateway Out23/1 -> To Workspace32/1
  Gateway Out34/1 -> To Workspace45/1
  Gateway Out35/1 -> To Workspace46/1
  Gateway Out37/1 -> To Workspace47/1
  Gateway Out36/1 -> To Workspace48/1
  bus_expand7/8(lsb_out1) -> Gateway Out38/1
  bus_expand7/7(out2) -> Gateway Out39/1
  bus_expand7/6(out3) -> Gateway Out22/1
  bus_expand7/5(out4) -> Gateway Out23/1
  bus_expand7/4(out5) -> Gateway Out34/1
  bus_expand7/3(out6) -> Gateway Out35/1
  bus_expand7/2(out7) -> Gateway Out36/1
  bus_expand7/1(msb_out8) -> Gateway Out37/1
  [hmc_data_p0] -> bus_expand7/1(bus_in)
  Gateway Out59/1 -> To Workspace59/1
  [hmc_dvalid_p0] -> Gateway Out59/1
  Gateway Out60/1 -> To Workspace60/1
  [hmc_sync_p0] -> Gateway Out60/1
  Gateway Out62/1 -> To Workspace62/1
  Gateway Out63/1 -> To Workspace63/1
  Gateway Out70/1 -> To Workspace72/1
  Gateway Out71/1 -> To Workspace71/1
  Gateway Out64/1 -> To Workspace70/1
  Gateway Out65/1 -> To Workspace68/1
  Gateway Out66/1 -> To Workspace67/1
  Gateway Out67/1 -> To Workspace66/1
  Gateway Out69/1 -> To Workspace69/1
  Gateway Out68/1 -> To Workspace65/1
  bus_expand13/8(lsb_out1) -> Gateway Out70/1
  bus_expand13/7(out2) -> Gateway Out71/1
  bus_expand13/6(out3) -> Gateway Out64/1
  bus_expand13/5(out4) -> Gateway Out65/1
  bus_expand13/4(out5) -> Gateway Out66/1
  bus_expand13/3(out6) -> Gateway Out67/1
  bus_expand13/2(out7) -> Gateway Out68/1
  bus_expand13/1(msb_out8) -> Gateway Out69/1
  [cd_in] -> bus_expand13/1(bus_in), pipeline11/1(d)
  Constant14/1 -> Concat1/2
  Constant12/1 -> Concat1/1
  bus_expand5/8(lsb_out1) -> Gateway Out14/1
  bus_expand5/7(out2) -> Gateway Out16/1
  bus_expand5/6(out3) -> Gateway Out17/1
  bus_expand5/5(out4) -> Gateway Out10/1
  bus_expand5/4(out5) -> Gateway Out11/1
  bus_expand5/3(out6) -> Gateway Out20/1
  bus_expand5/2(out7) -> Gateway Out21/1
  bus_expand5/1(msb_out8) -> Gateway Out13/1
  [delay_d0] -> bus_expand5/1(bus_in)
  Gateway Out13/1 -> To Workspace30/1
  Gateway Out21/1 -> To Workspace6/1
  Gateway Out20/1 -> To Workspace7/1
  Gateway Out11/1 -> To Workspace8/1
  Gateway Out10/1 -> To Workspace15/1
  Gateway Out17/1 -> To Workspace24/1
  Gateway Out16/1 -> To Workspace29/1
  Gateway Out14/1 -> To Workspace25/1
  Gateway Out58/1 -> To Workspace58/1
  [delay_dv] -> Gateway Out58/1
  Gateway Out61/1 -> To Workspace61/1
  [delay_sync] -> Gateway Out61/1
  Gateway Out41/1 -> To Workspace51/1
  Gateway Out42/1 -> To Workspace52/1
  Gateway Out44/1 -> To Workspace53/1
  Gateway Out52/1 -> To Workspace54/1
  Gateway Out53/1 -> To Workspace55/1
  Gateway Out54/1 -> To Workspace56/1
  Gateway Out55/1 -> To Workspace57/1
  Gateway Out56/1 -> To Workspace64/1
  Gateway Out57/1 -> To Workspace73/1
  [data_tl_bs0] -> Gateway Out57/1, wb_prog_delay/3(din)
  Gateway Out72/1 -> To Workspace74/1
  Gateway Out73/1 -> To Workspace75/1
  Gateway Out74/1 -> To Workspace76/1
  pipeline31/1(q) -> Gateway Out75/1, bus_create1/1(in1)
  pipeline32/1(q) -> bus_create1/2(in2)
  pipeline33/1(q) -> bus_create1/3(in3)
  pipeline34/1(q) -> bus_create1/4(in4)
  pipeline35/1(q) -> bus_create1/5(in5)
  pipeline36/1(q) -> bus_create1/6(in6)
  pipeline37/1(q) -> bus_create1/7(in7)
  pipeline40/1(q) -> bus_create1/8(in8)
  Gateway Out75/1 -> To Workspace77/1
  bus_expand6/1(msb_out8) -> pipeline21/1(d)  "hmc_out9"
  bus_expand6/8(lsb_out1) -> pipeline42/1(d)  "hmc_out16"
  pipeline42/1(q) -> cd_out/8(in_d07)
  pipeline41/1(q) -> cd_out/7(in_d06)
  pipeline26/1(q) -> cd_out/6(in_d05)
  pipeline25/1(q) -> cd_out/5(in_d04)
  pipeline24/1(q) -> cd_out/4(in_d03)
  pipeline23/1(q) -> cd_out/3(in_d02)
  pipeline22/1(q) -> cd_out/2(in_d01)
  pipeline21/1(q) -> cd_out/1(in_d00)
  bus_expand6/7(out2) -> pipeline41/1(d)
  bus_expand6/5(out4) -> pipeline25/1(d)
  bus_expand6/4(out5) -> pipeline24/1(d)
  bus_expand6/6(out3) -> pipeline26/1(d)
  bus_expand6/3(out6) -> pipeline23/1(d)
  bus_expand6/2(out7) -> pipeline22/1(d)
  pipeline46/1(q) -> cd_out/9(in_dvalid)
  pipeline45/1(q) -> cd_out/10(in_sync)
  pipeline79/1(q) -> cd_out/12(trig)
  pipeline48/1(q) -> cd_out/11(we)
  Logical3/1 -> pipeline48/1(d)
  [delay_sync] -> pipeline45/1(d), Logical3/2, pipeline79/1(d)
  [delay_d0] -> bus_expand6/1(bus_in)
  [delay_dv] -> Logical3/1, pipeline46/1(d)
  bus_expand8/1(msb_out8) -> pipeline80/1(d)  "hmc_out9"
  bus_expand8/8(lsb_out1) -> pipeline89/1(d)  "hmc_out16"
  pipeline89/1(q) -> delay_tl_out/8(in_d07)
  pipeline88/1(q) -> delay_tl_out/7(in_d06)
  pipeline86/1(q) -> delay_tl_out/6(in_d05)
  pipeline85/1(q) -> delay_tl_out/5(in_d04)
  pipeline84/1(q) -> delay_tl_out/4(in_d03)
  pipeline83/1(q) -> delay_tl_out/3(in_d02)
  pipeline82/1(q) -> delay_tl_out/2(in_d01)
  pipeline80/1(q) -> delay_tl_out/1(in_d00)
  bus_expand8/7(out2) -> pipeline88/1(d)
  bus_expand8/5(out4) -> pipeline85/1(d)
  bus_expand8/4(out5) -> pipeline84/1(d)
  bus_expand8/6(out3) -> pipeline86/1(d)
  bus_expand8/3(out6) -> pipeline83/1(d)
  bus_expand8/2(out7) -> pipeline82/1(d)
  pipeline100/1(q) -> delay_tl_out/9(in_dvalid)
  pipeline90/1(q) -> delay_tl_out/10(in_sync)
  pipeline120/1(q) -> delay_tl_out/12(trig)
  pipeline119/1(q) -> delay_tl_out/11(we)
  Logical4/1 -> pipeline119/1(d)
  [delay_tl_sync0] -> pipeline90/1(d), Logical4/2, pipeline120/1(d)
  [data_tl_bs0] -> bus_expand8/1(bus_in)
  [dvalid_tl_bs0] -> Logical4/1, pipeline100/1(d)
  Gateway Out82/1 -> To Workspace85/1
  Gateway Out83/1 -> To Workspace78/1
  Gateway Out76/1 -> To Workspace79/1
  Gateway Out77/1 -> To Workspace80/1
  Gateway Out78/1 -> To Workspace81/1
  Gateway Out79/1 -> To Workspace82/1
  Gateway Out81/1 -> To Workspace83/1
  Gateway Out80/1 -> To Workspace84/1
  bus_expand9/8(lsb_out1) -> Gateway Out82/1
  bus_expand9/7(out2) -> Gateway Out83/1
  bus_expand9/6(out3) -> Gateway Out76/1
  bus_expand9/5(out4) -> Gateway Out77/1
  bus_expand9/4(out5) -> Gateway Out78/1
  bus_expand9/3(out6) -> Gateway Out79/1
  bus_expand9/2(out7) -> Gateway Out80/1
  bus_expand9/1(msb_out8) -> Gateway Out81/1
  [data_tl_bs0] -> bus_expand9/1(bus_in)
  [hmc_data_p0] -> Delay20/1
  Delay20/1 -> [tg_data_p0]
  [tg_data_p0] -> pipeline117/1(d)
